simulink model "w3_warplab_trigger_proc"  (Simulink 7.7)
settings: Solver=ode45  StartTime=0.0  StopTime=60  RelTol=1e-3
InitFcn:
  | w3_warplab_trigger_proc_init
StartFcn:
  | w3_warplab_trigger_proc_init
undefined symbols (not defined in the file): gcbh, xlBlockLoadCallback, xlGetNormalizedPeriod
libraries: xbsIndex_r4 x1289, xbsEDKLib_r4 x1, simulink x1
(part 9 of 10)

== system w3_warplab_trigger_proc/Trigger Sources/Energy/AntC Detector/Busy Detection/S-R Latch ==
  R : Inport
  S : Inport  Port=2
  Constant1 : xbsIndex_r4/Constant  const=1  gui_display_data_type=Fixed-point  arith_type=Boolean  n_bits=1  bin_pt=0  preci_type=Single  exp_width=8  frac_width=24  explicit_period=off  period=1  equ=P=C  opselect=C  inp2=PCIN>>17  opr=+  inp1=P  carry=CIN  dbl_ovrd=off  block_type=constant
      settings: block_version=VER_STRING_GOES_HERE
  Register2 : xbsIndex_r4/Register  init=0  rst=on  en=on  dbl_ovrd=off  block_type=register
      settings: xl_area=[1 1 0 0 0 0 0]  block_version=VER_STRING_GOES_HERE
  Q : Outport
  wires:
  Constant1/1 -> Register2/1
  R/1 -> Register2/2
  Register2/1 -> Q/1
  S/1 -> Register2/3

== system w3_warplab_trigger_proc/Trigger Sources/Energy/AntC Detector/Idle Detection/S-R Latch ==
  R : Inport
  S : Inport  Port=2
  Constant1 : xbsIndex_r4/Constant  const=1  gui_display_data_type=Fixed-point  arith_type=Boolean  n_bits=1  bin_pt=0  preci_type=Single  exp_width=8  frac_width=24  explicit_period=off  period=1  equ=P=C  opselect=C  inp2=PCIN>>17  opr=+  inp1=P  carry=CIN  dbl_ovrd=off  block_type=constant
      settings: block_version=VER_STRING_GOES_HERE
  Register2 : xbsIndex_r4/Register  init=0  rst=on  en=on  dbl_ovrd=off  block_type=register
      settings: xl_area=[1 1 0 0 0 0 0]  block_version=VER_STRING_GOES_HERE
  Q : Outport
  wires:
  S/1 -> Register2/3
  Register2/1 -> Q/1
  R/1 -> Register2/2
  Constant1/1 -> Register2/1

== system w3_warplab_trigger_proc/Trigger Sources/Energy/AntC Detector/Running Sum/Long Reset Gen ==
  duration : Inport
  reset_in : Inport  Port=2
  Counter : xbsIndex_r4/Counter  cnt_type=Free Running  cnt_to=0  operation=Up  start_count=0  cnt_by_val=1  arith_type=Unsigned  n_bits=8  bin_pt=0  load_pin=off  rst=on  en=on  explicit_period=off  period=4  dbl_ovrd=off  use_behavioral_HDL=off  implementation=Fabric  use_rpm=off  block_type=counter
      settings: block_version=VER_STRING_GOES_HERE
  Relational : xbsIndex_r4/Relational  mode=a=b  en=off  latency=0  dbl_ovrd=off  block_type=relational
      settings: block_version=VER_STRING_GOES_HERE
  S-R Latch : Subsystem
  reset_out : Outport
  wires:
  Relational/1 -> Counter/1, S-R Latch/2(R)
  Counter/1 -> Relational/1
  reset_in/1 -> S-R Latch/1(S)
  duration/1 -> Relational/2
  S-R Latch/1(Q) -> Counter/2, reset_out/1

== system w3_warplab_trigger_proc/Trigger Sources/Energy/AntD Detector/Busy Detection/S-R Latch ==
  R : Inport
  S : Inport  Port=2
  Constant1 : xbsIndex_r4/Constant  const=1  gui_display_data_type=Fixed-point  arith_type=Boolean  n_bits=1  bin_pt=0  preci_type=Single  exp_width=8  frac_width=24  explicit_period=off  period=1  equ=P=C  opselect=C  inp2=PCIN>>17  opr=+  inp1=P  carry=CIN  dbl_ovrd=off  block_type=constant
      settings: block_version=VER_STRING_GOES_HERE
  Register2 : xbsIndex_r4/Register  init=0  rst=on  en=on  dbl_ovrd=off  block_type=register
      settings: xl_area=[1 1 0 0 0 0 0]  block_version=VER_STRING_GOES_HERE
  Q : Outport
  wires:
  Constant1/1 -> Register2/1
  R/1 -> Register2/2
  Register2/1 -> Q/1
  S/1 -> Register2/3

== system w3_warplab_trigger_proc/Trigger Sources/Energy/AntD Detector/Idle Detection/S-R Latch ==
  R : Inport
  S : Inport  Port=2
  Constant1 : xbsIndex_r4/Constant  const=1  gui_display_data_type=Fixed-point  arith_type=Boolean  n_bits=1  bin_pt=0  preci_type=Single  exp_width=8  frac_width=24  explicit_period=off  period=1  equ=P=C  opselect=C  inp2=PCIN>>17  opr=+  inp1=P  carry=CIN  dbl_ovrd=off  block_type=constant
      settings: block_version=VER_STRING_GOES_HERE
  Register2 : xbsIndex_r4/Register  init=0  rst=on  en=on  dbl_ovrd=off  block_type=register
      settings: xl_area=[1 1 0 0 0 0 0]  block_version=VER_STRING_GOES_HERE
  Q : Outport
  wires:
  S/1 -> Register2/3
  Register2/1 -> Q/1
  R/1 -> Register2/2
  Constant1/1 -> Register2/1

== system w3_warplab_trigger_proc/Trigger Sources/Energy/AntD Detector/Running Sum/Long Reset Gen ==
  duration : Inport
  reset_in : Inport  Port=2
  Counter : xbsIndex_r4/Counter  cnt_type=Free Running  cnt_to=0  operation=Up  start_count=0  cnt_by_val=1  arith_type=Unsigned  n_bits=8  bin_pt=0  load_pin=off  rst=on  en=on  explicit_period=off  period=4  dbl_ovrd=off  use_behavioral_HDL=off  implementation=Fabric  use_rpm=off  block_type=counter
      settings: block_version=VER_STRING_GOES_HERE
  Relational : xbsIndex_r4/Relational  mode=a=b  en=off  latency=0  dbl_ovrd=off  block_type=relational
      settings: block_version=VER_STRING_GOES_HERE
  S-R Latch : Subsystem
  reset_out : Outport
  wires:
  S-R Latch/1(Q) -> reset_out/1, Counter/2
  duration/1 -> Relational/2
  reset_in/1 -> S-R Latch/1(S)
  Counter/1 -> Relational/1
  Relational/1 -> S-R Latch/2(R), Counter/1

== system w3_warplab_trigger_proc/Trigger Sources/Ethernet A/Pkt Comp/Pkt Match 0/Pkt Match Fail ==
  S : Inport
  R : Inport  Port=2
  Constant5 : xbsIndex_r4/Constant  const=1  gui_display_data_type=Fixed-point  arith_type=Unsigned  n_bits=1  bin_pt=0  preci_type=Single  exp_width=8  frac_width=24  explicit_period=off  period=1  equ=P=C  opselect=C  inp2=PCIN>>17  opr=+  inp1=P  carry=CIN  dbl_ovrd=off  block_type=constant
  Convert : xbsIndex_r4/Convert  gui_display_data_type=Boolean  arith_type=Boolean  n_bits=16  bin_pt=14  float_type=Single  exp_bits=8  fraction_bits=24  quantization=Truncate  overflow=Wrap  en=off  latency=0  dbl_ovrd=off  pipeline=off  block_type=convert
  Convert1 : xbsIndex_r4/Convert  gui_display_data_type=Boolean  arith_type=Boolean  n_bits=16  bin_pt=14  float_type=Single  exp_bits=8  fraction_bits=24  quantization=Truncate  overflow=Wrap  en=off  latency=0  dbl_ovrd=off  pipeline=off  block_type=convert
  Register : xbsIndex_r4/Register  init=0  rst=on  en=on  dbl_ovrd=off  block_type=register
  Q : Outport
  wires:
  Constant5/1 -> Register/1
  R/1 -> Convert/1
  Register/1 -> Q/1
  S/1 -> Convert1/1
  Convert/1 -> Register/2
  Convert1/1 -> Register/3

== system w3_warplab_trigger_proc/Trigger Sources/Ethernet A/Pkt Comp/Word Comp 0/Byte Comp 0 ==
  note: Valid Op Codes:
      | 0: Don't care (always match)
      | 1: Equal (all bits match)
      | 2: Not-equal (>0 bits don't match)
      | 3: Any bit matches (AND(T,D)>0)
  Data : Inport
  Op : Inport  Port=2
  Template : Inport  Port=3
  2LSB : xbsIndex_r4/Slice  nbits=2  boolean_output=off  mode=Lower Bit Location + Width  bit1=0  base1=MSB of Input  bit0=0  base0=LSB of Input  dbl_ovrd=off  block_type=slice
  Any of AND : Subsystem
  Constant : xbsIndex_r4/Constant  const=1  gui_display_data_type=Boolean  arith_type=Boolean  n_bits=16  bin_pt=14  preci_type=Single  exp_width=8  frac_width=24  explicit_period=off  period=1  equ=P=C  opselect=C  inp2=PCIN>>17  opr=+  inp1=P  carry=CIN  dbl_ovrd=off  block_type=constant
  Constant1 : xbsIndex_r4/Constant  const=0  gui_display_data_type=Fixed-point  arith_type=Unsigned  n_bits=1  bin_pt=0  preci_type=Single  exp_width=8  frac_width=24  explicit_period=off  period=1  equ=P=C  opselect=C  inp2=PCIN>>17  opr=+  inp1=P  carry=CIN  dbl_ovrd=off  block_type=constant
  Constant2 : xbsIndex_r4/Constant  const=0  gui_display_data_type=Fixed-point  arith_type=Unsigned  n_bits=1  bin_pt=0  preci_type=Single  exp_width=8  frac_width=24  explicit_period=off  period=1  equ=P=C  opselect=C  inp2=PCIN>>17  opr=+  inp1=P  carry=CIN  dbl_ovrd=off  block_type=constant
  Constant3 : xbsIndex_r4/Constant  const=0  gui_display_data_type=Fixed-point  arith_type=Unsigned  n_bits=1  bin_pt=0  preci_type=Single  exp_width=8  frac_width=24  explicit_period=off  period=1  equ=P=C  opselect=C  inp2=PCIN>>17  opr=+  inp1=P  carry=CIN  dbl_ovrd=off  block_type=constant
  Constant4 : xbsIndex_r4/Constant  const=1  gui_display_data_type=Fixed-point  arith_type=Unsigned  n_bits=1  bin_pt=0  preci_type=Single  exp_width=8  frac_width=24  explicit_period=off  period=1  equ=P=C  opselect=C  inp2=PCIN>>17  opr=+  inp1=P  carry=CIN  dbl_ovrd=off  block_type=constant
  Equal : Subsystem
  Mux : xbsIndex_r4/Mux  inputs=4  en=off  latency=0  precision=Full  arith_type=Unsigned  n_bits=16  bin_pt=14  quantization=Truncate  overflow=Wrap  dbl_ovrd=off  block_type=mux
  Mux1 : xbsIndex_r4/Mux  inputs=4  en=off  latency=0  precision=Full  arith_type=Unsigned  n_bits=16  bin_pt=14  quantization=Truncate  overflow=Wrap  dbl_ovrd=off  block_type=mux
  Not Equal : Subsystem
  Res : Outport
  Or Op : Outport  Port=2
  wires:
  Op/1 -> 2LSB/1
  Mux/1 -> Res/1
  Constant/1 -> Mux/2
  Equal/1(R) -> Mux/3
  Not Equal/1(R) -> Mux/4
  Any of AND/1(R) -> Mux/5
  Data/1 -> Equal/1(D), Not Equal/1(D), Any of AND/1(D)
  Template/1 -> Equal/2(BT), Not Equal/2(BT), Any of AND/2(T)
  2LSB/1 -> Mux/1, Mux1/1
  Mux1/1 -> Or Op/1
  Constant1/1 -> Mux1/2
  Constant2/1 -> Mux1/3
  Constant3/1 -> Mux1/4
  Constant4/1 -> Mux1/5

== system w3_warplab_trigger_proc/Trigger Sources/Ethernet A/Pkt Comp/Word Comp 0/Byte Comp 1 ==
  note: Valid Op Codes:
      | 0: Don't care (always match)
      | 1: Equal (all bits match)
      | 2: Not-equal (>0 bits don't match)
      | 3: Any bit matches (AND(T,D)>0)
  Data : Inport
  Op : Inport  Port=2
  Template : Inport  Port=3
  2LSB : xbsIndex_r4/Slice  nbits=2  boolean_output=off  mode=Lower Bit Location + Width  bit1=0  base1=MSB of Input  bit0=0  base0=LSB of Input  dbl_ovrd=off  block_type=slice
  Any of AND : Subsystem
  Constant : xbsIndex_r4/Constant  const=1  gui_display_data_type=Boolean  arith_type=Boolean  n_bits=16  bin_pt=14  preci_type=Single  exp_width=8  frac_width=24  explicit_period=off  period=1  equ=P=C  opselect=C  inp2=PCIN>>17  opr=+  inp1=P  carry=CIN  dbl_ovrd=off  block_type=constant
  Constant1 : xbsIndex_r4/Constant  const=0  gui_display_data_type=Fixed-point  arith_type=Unsigned  n_bits=1  bin_pt=0  preci_type=Single  exp_width=8  frac_width=24  explicit_period=off  period=1  equ=P=C  opselect=C  inp2=PCIN>>17  opr=+  inp1=P  carry=CIN  dbl_ovrd=off  block_type=constant
  Constant2 : xbsIndex_r4/Constant  const=0  gui_display_data_type=Fixed-point  arith_type=Unsigned  n_bits=1  bin_pt=0  preci_type=Single  exp_width=8  frac_width=24  explicit_period=off  period=1  equ=P=C  opselect=C  inp2=PCIN>>17  opr=+  inp1=P  carry=CIN  dbl_ovrd=off  block_type=constant
  Constant3 : xbsIndex_r4/Constant  const=0  gui_display_data_type=Fixed-point  arith_type=Unsigned  n_bits=1  bin_pt=0  preci_type=Single  exp_width=8  frac_width=24  explicit_period=off  period=1  equ=P=C  opselect=C  inp2=PCIN>>17  opr=+  inp1=P  carry=CIN  dbl_ovrd=off  block_type=constant
  Constant4 : xbsIndex_r4/Constant  const=1  gui_display_data_type=Fixed-point  arith_type=Unsigned  n_bits=1  bin_pt=0  preci_type=Single  exp_width=8  frac_width=24  explicit_period=off  period=1  equ=P=C  opselect=C  inp2=PCIN>>17  opr=+  inp1=P  carry=CIN  dbl_ovrd=off  block_type=constant
  Equal : Subsystem
  Mux : xbsIndex_r4/Mux  inputs=4  en=off  latency=0  precision=Full  arith_type=Unsigned  n_bits=16  bin_pt=14  quantization=Truncate  overflow=Wrap  dbl_ovrd=off  block_type=mux
  Mux1 : xbsIndex_r4/Mux  inputs=4  en=off  latency=0  precision=Full  arith_type=Unsigned  n_bits=16  bin_pt=14  quantization=Truncate  overflow=Wrap  dbl_ovrd=off  block_type=mux
  Not Equal : Subsystem
  Res : Outport
  Or Op : Outport  Port=2
  wires:
  Constant4/1 -> Mux1/5
  Constant3/1 -> Mux1/4
  Constant2/1 -> Mux1/3
  Constant1/1 -> Mux1/2
  Mux1/1 -> Or Op/1
  2LSB/1 -> Mux1/1, Mux/1
  Template/1 -> Any of AND/2(T), Not Equal/2(BT), Equal/2(BT)
  Data/1 -> Any of AND/1(D), Not Equal/1(D), Equal/1(D)
  Any of AND/1(R) -> Mux/5
  Not Equal/1(R) -> Mux/4
  Equal/1(R) -> Mux/3
  Constant/1 -> Mux/2
  Mux/1 -> Res/1
  Op/1 -> 2LSB/1

== system w3_warplab_trigger_proc/Trigger Sources/Ethernet A/Pkt Comp/Word Comp 0/Byte Comp 2 ==
  note: Valid Op Codes:
      | 0: Don't care (always match)
      | 1: Equal (all bits match)
      | 2: Not-equal (>0 bits don't match)
      | 3: Any bit matches (AND(T,D)>0)
  Data : Inport
  Op : Inport  Port=2
  Template : Inport  Port=3
  2LSB : xbsIndex_r4/Slice  nbits=2  boolean_output=off  mode=Lower Bit Location + Width  bit1=0  base1=MSB of Input  bit0=0  base0=LSB of Input  dbl_ovrd=off  block_type=slice
  Any of AND : Subsystem
  Constant : xbsIndex_r4/Constant  const=1  gui_display_data_type=Boolean  arith_type=Boolean  n_bits=16  bin_pt=14  preci_type=Single  exp_width=8  frac_width=24  explicit_period=off  period=1  equ=P=C  opselect=C  inp2=PCIN>>17  opr=+  inp1=P  carry=CIN  dbl_ovrd=off  block_type=constant
  Constant1 : xbsIndex_r4/Constant  const=0  gui_display_data_type=Fixed-point  arith_type=Unsigned  n_bits=1  bin_pt=0  preci_type=Single  exp_width=8  frac_width=24  explicit_period=off  period=1  equ=P=C  opselect=C  inp2=PCIN>>17  opr=+  inp1=P  carry=CIN  dbl_ovrd=off  block_type=constant
  Constant2 : xbsIndex_r4/Constant  const=0  gui_display_data_type=Fixed-point  arith_type=Unsigned  n_bits=1  bin_pt=0  preci_type=Single  exp_width=8  frac_width=24  explicit_period=off  period=1  equ=P=C  opselect=C  inp2=PCIN>>17  opr=+  inp1=P  carry=CIN  dbl_ovrd=off  block_type=constant
  Constant3 : xbsIndex_r4/Constant  const=0  gui_display_data_type=Fixed-point  arith_type=Unsigned  n_bits=1  bin_pt=0  preci_type=Single  exp_width=8  frac_width=24  explicit_period=off  period=1  equ=P=C  opselect=C  inp2=PCIN>>17  opr=+  inp1=P  carry=CIN  dbl_ovrd=off  block_type=constant
  Constant4 : xbsIndex_r4/Constant  const=1  gui_display_data_type=Fixed-point  arith_type=Unsigned  n_bits=1  bin_pt=0  preci_type=Single  exp_width=8  frac_width=24  explicit_period=off  period=1  equ=P=C  opselect=C  inp2=PCIN>>17  opr=+  inp1=P  carry=CIN  dbl_ovrd=off  block_type=constant
  Equal : Subsystem
  Mux : xbsIndex_r4/Mux  inputs=4  en=off  latency=0  precision=Full  arith_type=Unsigned  n_bits=16  bin_pt=14  quantization=Truncate  overflow=Wrap  dbl_ovrd=off  block_type=mux
  Mux1 : xbsIndex_r4/Mux  inputs=4  en=off  latency=0  precision=Full  arith_type=Unsigned  n_bits=16  bin_pt=14  quantization=Truncate  overflow=Wrap  dbl_ovrd=off  block_type=mux
  Not Equal : Subsystem
  Res : Outport
  Or Op : Outport  Port=2
  wires:
  Op/1 -> 2LSB/1
  Mux/1 -> Res/1
  Constant/1 -> Mux/2
  Equal/1(R) -> Mux/3
  Not Equal/1(R) -> Mux/4
  Any of AND/1(R) -> Mux/5
  Data/1 -> Equal/1(D), Not Equal/1(D), Any of AND/1(D)
  Template/1 -> Equal/2(BT), Not Equal/2(BT), Any of AND/2(T)
  2LSB/1 -> Mux/1, Mux1/1
  Mux1/1 -> Or Op/1
  Constant1/1 -> Mux1/2
  Constant2/1 -> Mux1/3
  Constant3/1 -> Mux1/4
  Constant4/1 -> Mux1/5

== system w3_warplab_trigger_proc/Trigger Sources/Ethernet A/Pkt Comp/Word Comp 0/Byte Comp 3 ==
  note: Valid Op Codes:
      | 0: Don't care (always match)
      | 1: Equal (all bits match)
      | 2: Not-equal (>0 bits don't match)
      | 3: Any bit matches (AND(T,D)>0)
  Data : Inport
  Op : Inport  Port=2
  Template : Inport  Port=3
  2LSB : xbsIndex_r4/Slice  nbits=2  boolean_output=off  mode=Lower Bit Location + Width  bit1=0  base1=MSB of Input  bit0=0  base0=LSB of Input  dbl_ovrd=off  block_type=slice
  Any of AND : Subsystem
  Constant : xbsIndex_r4/Constant  const=1  gui_display_data_type=Boolean  arith_type=Boolean  n_bits=16  bin_pt=14  preci_type=Single  exp_width=8  frac_width=24  explicit_period=off  period=1  equ=P=C  opselect=C  inp2=PCIN>>17  opr=+  inp1=P  carry=CIN  dbl_ovrd=off  block_type=constant
  Constant1 : xbsIndex_r4/Constant  const=0  gui_display_data_type=Fixed-point  arith_type=Unsigned  n_bits=1  bin_pt=0  preci_type=Single  exp_width=8  frac_width=24  explicit_period=off  period=1  equ=P=C  opselect=C  inp2=PCIN>>17  opr=+  inp1=P  carry=CIN  dbl_ovrd=off  block_type=constant
  Constant2 : xbsIndex_r4/Constant  const=0  gui_display_data_type=Fixed-point  arith_type=Unsigned  n_bits=1  bin_pt=0  preci_type=Single  exp_width=8  frac_width=24  explicit_period=off  period=1  equ=P=C  opselect=C  inp2=PCIN>>17  opr=+  inp1=P  carry=CIN  dbl_ovrd=off  block_type=constant
  Constant3 : xbsIndex_r4/Constant  const=0  gui_display_data_type=Fixed-point  arith_type=Unsigned  n_bits=1  bin_pt=0  preci_type=Single  exp_width=8  frac_width=24  explicit_period=off  period=1  equ=P=C  opselect=C  inp2=PCIN>>17  opr=+  inp1=P  carry=CIN  dbl_ovrd=off  block_type=constant
  Constant4 : xbsIndex_r4/Constant  const=1  gui_display_data_type=Fixed-point  arith_type=Unsigned  n_bits=1  bin_pt=0  preci_type=Single  exp_width=8  frac_width=24  explicit_period=off  period=1  equ=P=C  opselect=C  inp2=PCIN>>17  opr=+  inp1=P  carry=CIN  dbl_ovrd=off  block_type=constant
  Equal : Subsystem
  Mux : xbsIndex_r4/Mux  inputs=4  en=off  latency=0  precision=Full  arith_type=Unsigned  n_bits=16  bin_pt=14  quantization=Truncate  overflow=Wrap  dbl_ovrd=off  block_type=mux
  Mux1 : xbsIndex_r4/Mux  inputs=4  en=off  latency=0  precision=Full  arith_type=Unsigned  n_bits=16  bin_pt=14  quantization=Truncate  overflow=Wrap  dbl_ovrd=off  block_type=mux
  Not Equal : Subsystem
  Res : Outport
  Or Op : Outport  Port=2
  wires:
  Constant4/1 -> Mux1/5
  Constant3/1 -> Mux1/4
  Constant2/1 -> Mux1/3
  Constant1/1 -> Mux1/2
  Mux1/1 -> Or Op/1
  2LSB/1 -> Mux1/1, Mux/1
  Template/1 -> Any of AND/2(T), Not Equal/2(BT), Equal/2(BT)
  Data/1 -> Any of AND/1(D), Not Equal/1(D), Equal/1(D)
  Any of AND/1(R) -> Mux/5
  Not Equal/1(R) -> Mux/4
  Equal/1(R) -> Mux/3
  Constant/1 -> Mux/2
  Mux/1 -> Res/1
  Op/1 -> 2LSB/1

== system w3_warplab_trigger_proc/Trigger Sources/Ethernet A/Pkt Comp/Word Comp 0/Subsystem ==
  32b : Inport
  8LSB+0 : xbsIndex_r4/Slice  nbits=8  boolean_output=off  mode=Lower Bit Location + Width  bit1=0  base1=MSB of Input  bit0=0  base0=LSB of Input  dbl_ovrd=off  block_type=slice
  8LSB+16 : xbsIndex_r4/Slice  nbits=8  boolean_output=off  mode=Lower Bit Location + Width  bit1=0  base1=MSB of Input  bit0=16  base0=LSB of Input  dbl_ovrd=off  block_type=slice
  8LSB+24 : xbsIndex_r4/Slice  nbits=8  boolean_output=off  mode=Lower Bit Location + Width  bit1=0  base1=MSB of Input  bit0=24  base0=LSB of Input  dbl_ovrd=off  block_type=slice
  8LSB+8 : xbsIndex_r4/Slice  nbits=8  boolean_output=off  mode=Lower Bit Location + Width  bit1=0  base1=MSB of Input  bit0=8  base0=LSB of Input  dbl_ovrd=off  block_type=slice
  B0 : Outport
  B1 : Outport  Port=2
  B2 : Outport  Port=3
  B3 : Outport  Port=4
  wires:
  32b/1 -> 8LSB+0/1, 8LSB+8/1, 8LSB+16/1, 8LSB+24/1
  8LSB+0/1 -> B0/1
  8LSB+8/1 -> B1/1
  8LSB+16/1 -> B2/1
  8LSB+24/1 -> B3/1

== system w3_warplab_trigger_proc/Trigger Sources/Ethernet A/Pkt Comp/Word Comp 0/Subsystem1 ==
  32b : Inport
  8LSB+0 : xbsIndex_r4/Slice  nbits=8  boolean_output=off  mode=Lower Bit Location + Width  bit1=0  base1=MSB of Input  bit0=0  base0=LSB of Input  dbl_ovrd=off  block_type=slice
  8LSB+16 : xbsIndex_r4/Slice  nbits=8  boolean_output=off  mode=Lower Bit Location + Width  bit1=0  base1=MSB of Input  bit0=16  base0=LSB of Input  dbl_ovrd=off  block_type=slice
  8LSB+24 : xbsIndex_r4/Slice  nbits=8  boolean_output=off  mode=Lower Bit Location + Width  bit1=0  base1=MSB of Input  bit0=24  base0=LSB of Input  dbl_ovrd=off  block_type=slice
  8LSB+8 : xbsIndex_r4/Slice  nbits=8  boolean_output=off  mode=Lower Bit Location + Width  bit1=0  base1=MSB of Input  bit0=8  base0=LSB of Input  dbl_ovrd=off  block_type=slice
  B0 : Outport
  B1 : Outport  Port=2
  B2 : Outport  Port=3
  B3 : Outport  Port=4
  wires:
  8LSB+24/1 -> B3/1
  8LSB+16/1 -> B2/1
  8LSB+8/1 -> B1/1
  8LSB+0/1 -> B0/1
  32b/1 -> 8LSB+24/1, 8LSB+16/1, 8LSB+8/1, 8LSB+0/1

== system w3_warplab_trigger_proc/Trigger Sources/Ethernet A/Pkt Comp/Word Comp 0/Subsystem2 ==
  32b : Inport
  8LSB+0 : xbsIndex_r4/Slice  nbits=8  boolean_output=off  mode=Lower Bit Location + Width  bit1=0  base1=MSB of Input  bit0=0  base0=LSB of Input  dbl_ovrd=off  block_type=slice
  8LSB+16 : xbsIndex_r4/Slice  nbits=8  boolean_output=off  mode=Lower Bit Location + Width  bit1=0  base1=MSB of Input  bit0=16  base0=LSB of Input  dbl_ovrd=off  block_type=slice
  8LSB+24 : xbsIndex_r4/Slice  nbits=8  boolean_output=off  mode=Lower Bit Location + Width  bit1=0  base1=MSB of Input  bit0=24  base0=LSB of Input  dbl_ovrd=off  block_type=slice
  8LSB+8 : xbsIndex_r4/Slice  nbits=8  boolean_output=off  mode=Lower Bit Location + Width  bit1=0  base1=MSB of Input  bit0=8  base0=LSB of Input  dbl_ovrd=off  block_type=slice
  B0 : Outport
  B1 : Outport  Port=2
  B2 : Outport  Port=3
  B3 : Outport  Port=4
  wires:
  32b/1 -> 8LSB+0/1, 8LSB+8/1, 8LSB+16/1, 8LSB+24/1
  8LSB+0/1 -> B0/1
  8LSB+8/1 -> B1/1
  8LSB+16/1 -> B2/1
  8LSB+24/1 -> B3/1

== system w3_warplab_trigger_proc/Trigger Sources/Ethernet B/Pkt Comp/Pkt Match 1/Pkt Match Fail ==
  S : Inport
  R : Inport  Port=2
  Constant5 : xbsIndex_r4/Constant  const=1  gui_display_data_type=Fixed-point  arith_type=Unsigned  n_bits=1  bin_pt=0  preci_type=Single  exp_width=8  frac_width=24  explicit_period=off  period=1  equ=P=C  opselect=C  inp2=PCIN>>17  opr=+  inp1=P  carry=CIN  dbl_ovrd=off  block_type=constant
  Convert : xbsIndex_r4/Convert  gui_display_data_type=Boolean  arith_type=Boolean  n_bits=16  bin_pt=14  float_type=Single  exp_bits=8  fraction_bits=24  quantization=Truncate  overflow=Wrap  en=off  latency=0  dbl_ovrd=off  pipeline=off  block_type=convert
  Convert1 : xbsIndex_r4/Convert  gui_display_data_type=Boolean  arith_type=Boolean  n_bits=16  bin_pt=14  float_type=Single  exp_bits=8  fraction_bits=24  quantization=Truncate  overflow=Wrap  en=off  latency=0  dbl_ovrd=off  pipeline=off  block_type=convert
  Register : xbsIndex_r4/Register  init=0  rst=on  en=on  dbl_ovrd=off  block_type=register
  Q : Outport
  wires:
  Constant5/1 -> Register/1
  R/1 -> Convert/1
  Register/1 -> Q/1
  S/1 -> Convert1/1
  Convert/1 -> Register/2
  Convert1/1 -> Register/3

== system w3_warplab_trigger_proc/Trigger Sources/Ethernet B/Pkt Comp/Word Comp 1/Byte Comp 0 ==
  note: Valid Op Codes:
      | 0: Don't care (always match)
      | 1: Equal (all bits match)
      | 2: Not-equal (>0 bits don't match)
      | 3: Any bit matches (AND(T,D)>0)
  Data : Inport
  Op : Inport  Port=2
  Template : Inport  Port=3
  2LSB : xbsIndex_r4/Slice  nbits=2  boolean_output=off  mode=Lower Bit Location + Width  bit1=0  base1=MSB of Input  bit0=0  base0=LSB of Input  dbl_ovrd=off  block_type=slice
  Any of AND : Subsystem
  Constant : xbsIndex_r4/Constant  const=1  gui_display_data_type=Boolean  arith_type=Boolean  n_bits=16  bin_pt=14  preci_type=Single  exp_width=8  frac_width=24  explicit_period=off  period=1  equ=P=C  opselect=C  inp2=PCIN>>17  opr=+  inp1=P  carry=CIN  dbl_ovrd=off  block_type=constant
  Constant1 : xbsIndex_r4/Constant  const=0  gui_display_data_type=Fixed-point  arith_type=Unsigned  n_bits=1  bin_pt=0  preci_type=Single  exp_width=8  frac_width=24  explicit_period=off  period=1  equ=P=C  opselect=C  inp2=PCIN>>17  opr=+  inp1=P  carry=CIN  dbl_ovrd=off  block_type=constant
  Constant2 : xbsIndex_r4/Constant  const=0  gui_display_data_type=Fixed-point  arith_type=Unsigned  n_bits=1  bin_pt=0  preci_type=Single  exp_width=8  frac_width=24  explicit_period=off  period=1  equ=P=C  opselect=C  inp2=PCIN>>17  opr=+  inp1=P  carry=CIN  dbl_ovrd=off  block_type=constant
  Constant3 : xbsIndex_r4/Constant  const=0  gui_display_data_type=Fixed-point  arith_type=Unsigned  n_bits=1  bin_pt=0  preci_type=Single  exp_width=8  frac_width=24  explicit_period=off  period=1  equ=P=C  opselect=C  inp2=PCIN>>17  opr=+  inp1=P  carry=CIN  dbl_ovrd=off  block_type=constant
  Constant4 : xbsIndex_r4/Constant  const=1  gui_display_data_type=Fixed-point  arith_type=Unsigned  n_bits=1  bin_pt=0  preci_type=Single  exp_width=8  frac_width=24  explicit_period=off  period=1  equ=P=C  opselect=C  inp2=PCIN>>17  opr=+  inp1=P  carry=CIN  dbl_ovrd=off  block_type=constant
  Equal : Subsystem
  Mux : xbsIndex_r4/Mux  inputs=4  en=off  latency=0  precision=Full  arith_type=Unsigned  n_bits=16  bin_pt=14  quantization=Truncate  overflow=Wrap  dbl_ovrd=off  block_type=mux
  Mux1 : xbsIndex_r4/Mux  inputs=4  en=off  latency=0  precision=Full  arith_type=Unsigned  n_bits=16  bin_pt=14  quantization=Truncate  overflow=Wrap  dbl_ovrd=off  block_type=mux
  Not Equal : Subsystem
  Res : Outport
  Or Op : Outport  Port=2
  wires:
  Op/1 -> 2LSB/1
  Mux/1 -> Res/1
  Constant/1 -> Mux/2
  Equal/1(R) -> Mux/3
  Not Equal/1(R) -> Mux/4
  Any of AND/1(R) -> Mux/5
  Data/1 -> Equal/1(D), Not Equal/1(D), Any of AND/1(D)
  Template/1 -> Equal/2(BT), Not Equal/2(BT), Any of AND/2(T)
  2LSB/1 -> Mux/1, Mux1/1
  Mux1/1 -> Or Op/1
  Constant1/1 -> Mux1/2
  Constant2/1 -> Mux1/3
  Constant3/1 -> Mux1/4
  Constant4/1 -> Mux1/5

== system w3_warplab_trigger_proc/Trigger Sources/Ethernet B/Pkt Comp/Word Comp 1/Byte Comp 1 ==
  note: Valid Op Codes:
      | 0: Don't care (always match)
      | 1: Equal (all bits match)
      | 2: Not-equal (>0 bits don't match)
      | 3: Any bit matches (AND(T,D)>0)
  Data : Inport
  Op : Inport  Port=2
  Template : Inport  Port=3
  2LSB : xbsIndex_r4/Slice  nbits=2  boolean_output=off  mode=Lower Bit Location + Width  bit1=0  base1=MSB of Input  bit0=0  base0=LSB of Input  dbl_ovrd=off  block_type=slice
  Any of AND : Subsystem
  Constant : xbsIndex_r4/Constant  const=1  gui_display_data_type=Boolean  arith_type=Boolean  n_bits=16  bin_pt=14  preci_type=Single  exp_width=8  frac_width=24  explicit_period=off  period=1  equ=P=C  opselect=C  inp2=PCIN>>17  opr=+  inp1=P  carry=CIN  dbl_ovrd=off  block_type=constant
  Constant1 : xbsIndex_r4/Constant  const=0  gui_display_data_type=Fixed-point  arith_type=Unsigned  n_bits=1  bin_pt=0  preci_type=Single  exp_width=8  frac_width=24  explicit_period=off  period=1  equ=P=C  opselect=C  inp2=PCIN>>17  opr=+  inp1=P  carry=CIN  dbl_ovrd=off  block_type=constant
  Constant2 : xbsIndex_r4/Constant  const=0  gui_display_data_type=Fixed-point  arith_type=Unsigned  n_bits=1  bin_pt=0  preci_type=Single  exp_width=8  frac_width=24  explicit_period=off  period=1  equ=P=C  opselect=C  inp2=PCIN>>17  opr=+  inp1=P  carry=CIN  dbl_ovrd=off  block_type=constant
  Constant3 : xbsIndex_r4/Constant  const=0  gui_display_data_type=Fixed-point  arith_type=Unsigned  n_bits=1  bin_pt=0  preci_type=Single  exp_width=8  frac_width=24  explicit_period=off  period=1  equ=P=C  opselect=C  inp2=PCIN>>17  opr=+  inp1=P  carry=CIN  dbl_ovrd=off  block_type=constant
  Constant4 : xbsIndex_r4/Constant  const=1  gui_display_data_type=Fixed-point  arith_type=Unsigned  n_bits=1  bin_pt=0  preci_type=Single  exp_width=8  frac_width=24  explicit_period=off  period=1  equ=P=C  opselect=C  inp2=PCIN>>17  opr=+  inp1=P  carry=CIN  dbl_ovrd=off  block_type=constant
  Equal : Subsystem
  Mux : xbsIndex_r4/Mux  inputs=4  en=off  latency=0  precision=Full  arith_type=Unsigned  n_bits=16  bin_pt=14  quantization=Truncate  overflow=Wrap  dbl_ovrd=off  block_type=mux
  Mux1 : xbsIndex_r4/Mux  inputs=4  en=off  latency=0  precision=Full  arith_type=Unsigned  n_bits=16  bin_pt=14  quantization=Truncate  overflow=Wrap  dbl_ovrd=off  block_type=mux
  Not Equal : Subsystem
  Res : Outport
  Or Op : Outport  Port=2
  wires:
  Constant4/1 -> Mux1/5
  Constant3/1 -> Mux1/4
  Constant2/1 -> Mux1/3
  Constant1/1 -> Mux1/2
  Mux1/1 -> Or Op/1
  2LSB/1 -> Mux1/1, Mux/1
  Template/1 -> Any of AND/2(T), Not Equal/2(BT), Equal/2(BT)
  Data/1 -> Any of AND/1(D), Not Equal/1(D), Equal/1(D)
  Any of AND/1(R) -> Mux/5
  Not Equal/1(R) -> Mux/4
  Equal/1(R) -> Mux/3
  Constant/1 -> Mux/2
  Mux/1 -> Res/1
  Op/1 -> 2LSB/1

== system w3_warplab_trigger_proc/Trigger Sources/Ethernet B/Pkt Comp/Word Comp 1/Byte Comp 2 ==
  note: Valid Op Codes:
      | 0: Don't care (always match)
      | 1: Equal (all bits match)
      | 2: Not-equal (>0 bits don't match)
      | 3: Any bit matches (AND(T,D)>0)
  Data : Inport
  Op : Inport  Port=2
  Template : Inport  Port=3
  2LSB : xbsIndex_r4/Slice  nbits=2  boolean_output=off  mode=Lower Bit Location + Width  bit1=0  base1=MSB of Input  bit0=0  base0=LSB of Input  dbl_ovrd=off  block_type=slice
  Any of AND : Subsystem
  Constant : xbsIndex_r4/Constant  const=1  gui_display_data_type=Boolean  arith_type=Boolean  n_bits=16  bin_pt=14  preci_type=Single  exp_width=8  frac_width=24  explicit_period=off  period=1  equ=P=C  opselect=C  inp2=PCIN>>17  opr=+  inp1=P  carry=CIN  dbl_ovrd=off  block_type=constant
  Constant1 : xbsIndex_r4/Constant  const=0  gui_display_data_type=Fixed-point  arith_type=Unsigned  n_bits=1  bin_pt=0  preci_type=Single  exp_width=8  frac_width=24  explicit_period=off  period=1  equ=P=C  opselect=C  inp2=PCIN>>17  opr=+  inp1=P  carry=CIN  dbl_ovrd=off  block_type=constant
  Constant2 : xbsIndex_r4/Constant  const=0  gui_display_data_type=Fixed-point  arith_type=Unsigned  n_bits=1  bin_pt=0  preci_type=Single  exp_width=8  frac_width=24  explicit_period=off  period=1  equ=P=C  opselect=C  inp2=PCIN>>17  opr=+  inp1=P  carry=CIN  dbl_ovrd=off  block_type=constant
  Constant3 : xbsIndex_r4/Constant  const=0  gui_display_data_type=Fixed-point  arith_type=Unsigned  n_bits=1  bin_pt=0  preci_type=Single  exp_width=8  frac_width=24  explicit_period=off  period=1  equ=P=C  opselect=C  inp2=PCIN>>17  opr=+  inp1=P  carry=CIN  dbl_ovrd=off  block_type=constant
  Constant4 : xbsIndex_r4/Constant  const=1  gui_display_data_type=Fixed-point  arith_type=Unsigned  n_bits=1  bin_pt=0  preci_type=Single  exp_width=8  frac_width=24  explicit_period=off  period=1  equ=P=C  opselect=C  inp2=PCIN>>17  opr=+  inp1=P  carry=CIN  dbl_ovrd=off  block_type=constant
  Equal : Subsystem
  Mux : xbsIndex_r4/Mux  inputs=4  en=off  latency=0  precision=Full  arith_type=Unsigned  n_bits=16  bin_pt=14  quantization=Truncate  overflow=Wrap  dbl_ovrd=off  block_type=mux
  Mux1 : xbsIndex_r4/Mux  inputs=4  en=off  latency=0  precision=Full  arith_type=Unsigned  n_bits=16  bin_pt=14  quantization=Truncate  overflow=Wrap  dbl_ovrd=off  block_type=mux
  Not Equal : Subsystem
  Res : Outport
  Or Op : Outport  Port=2
  wires:
  Op/1 -> 2LSB/1
  Mux/1 -> Res/1
  Constant/1 -> Mux/2
  Equal/1(R) -> Mux/3
  Not Equal/1(R) -> Mux/4
  Any of AND/1(R) -> Mux/5
  Data/1 -> Equal/1(D), Not Equal/1(D), Any of AND/1(D)
  Template/1 -> Equal/2(BT), Not Equal/2(BT), Any of AND/2(T)
  2LSB/1 -> Mux/1, Mux1/1
  Mux1/1 -> Or Op/1
  Constant1/1 -> Mux1/2
  Constant2/1 -> Mux1/3
  Constant3/1 -> Mux1/4
  Constant4/1 -> Mux1/5

== system w3_warplab_trigger_proc/Trigger Sources/Ethernet B/Pkt Comp/Word Comp 1/Byte Comp 3 ==
  note: Valid Op Codes:
      | 0: Don't care (always match)
      | 1: Equal (all bits match)
      | 2: Not-equal (>0 bits don't match)
      | 3: Any bit matches (AND(T,D)>0)
  Data : Inport
  Op : Inport  Port=2
  Template : Inport  Port=3
  2LSB : xbsIndex_r4/Slice  nbits=2  boolean_output=off  mode=Lower Bit Location + Width  bit1=0  base1=MSB of Input  bit0=0  base0=LSB of Input  dbl_ovrd=off  block_type=slice
  Any of AND : Subsystem
  Constant : xbsIndex_r4/Constant  const=1  gui_display_data_type=Boolean  arith_type=Boolean  n_bits=16  bin_pt=14  preci_type=Single  exp_width=8  frac_width=24  explicit_period=off  period=1  equ=P=C  opselect=C  inp2=PCIN>>17  opr=+  inp1=P  carry=CIN  dbl_ovrd=off  block_type=constant
  Constant1 : xbsIndex_r4/Constant  const=0  gui_display_data_type=Fixed-point  arith_type=Unsigned  n_bits=1  bin_pt=0  preci_type=Single  exp_width=8  frac_width=24  explicit_period=off  period=1  equ=P=C  opselect=C  inp2=PCIN>>17  opr=+  inp1=P  carry=CIN  dbl_ovrd=off  block_type=constant
  Constant2 : xbsIndex_r4/Constant  const=0  gui_display_data_type=Fixed-point  arith_type=Unsigned  n_bits=1  bin_pt=0  preci_type=Single  exp_width=8  frac_width=24  explicit_period=off  period=1  equ=P=C  opselect=C  inp2=PCIN>>17  opr=+  inp1=P  carry=CIN  dbl_ovrd=off  block_type=constant
  Constant3 : xbsIndex_r4/Constant  const=0  gui_display_data_type=Fixed-point  arith_type=Unsigned  n_bits=1  bin_pt=0  preci_type=Single  exp_width=8  frac_width=24  explicit_period=off  period=1  equ=P=C  opselect=C  inp2=PCIN>>17  opr=+  inp1=P  carry=CIN  dbl_ovrd=off  block_type=constant
  Constant4 : xbsIndex_r4/Constant  const=1  gui_display_data_type=Fixed-point  arith_type=Unsigned  n_bits=1  bin_pt=0  preci_type=Single  exp_width=8  frac_width=24  explicit_period=off  period=1  equ=P=C  opselect=C  inp2=PCIN>>17  opr=+  inp1=P  carry=CIN  dbl_ovrd=off  block_type=constant
  Equal : Subsystem
  Mux : xbsIndex_r4/Mux  inputs=4  en=off  latency=0  precision=Full  arith_type=Unsigned  n_bits=16  bin_pt=14  quantization=Truncate  overflow=Wrap  dbl_ovrd=off  block_type=mux
  Mux1 : xbsIndex_r4/Mux  inputs=4  en=off  latency=0  precision=Full  arith_type=Unsigned  n_bits=16  bin_pt=14  quantization=Truncate  overflow=Wrap  dbl_ovrd=off  block_type=mux
  Not Equal : Subsystem
  Res : Outport
  Or Op : Outport  Port=2
  wires:
  Constant4/1 -> Mux1/5
  Constant3/1 -> Mux1/4
  Constant2/1 -> Mux1/3
  Constant1/1 -> Mux1/2
  Mux1/1 -> Or Op/1
  2LSB/1 -> Mux1/1, Mux/1
  Template/1 -> Any of AND/2(T), Not Equal/2(BT), Equal/2(BT)
  Data/1 -> Any of AND/1(D), Not Equal/1(D), Equal/1(D)
  Any of AND/1(R) -> Mux/5
  Not Equal/1(R) -> Mux/4
  Equal/1(R) -> Mux/3
  Constant/1 -> Mux/2
  Mux/1 -> Res/1
  Op/1 -> 2LSB/1

== system w3_warplab_trigger_proc/Trigger Sources/Ethernet B/Pkt Comp/Word Comp 1/Subsystem ==
  32b : Inport
  8LSB+0 : xbsIndex_r4/Slice  nbits=8  boolean_output=off  mode=Lower Bit Location + Width  bit1=0  base1=MSB of Input  bit0=0  base0=LSB of Input  dbl_ovrd=off  block_type=slice
  8LSB+16 : xbsIndex_r4/Slice  nbits=8  boolean_output=off  mode=Lower Bit Location + Width  bit1=0  base1=MSB of Input  bit0=16  base0=LSB of Input  dbl_ovrd=off  block_type=slice
  8LSB+24 : xbsIndex_r4/Slice  nbits=8  boolean_output=off  mode=Lower Bit Location + Width  bit1=0  base1=MSB of Input  bit0=24  base0=LSB of Input  dbl_ovrd=off  block_type=slice
  8LSB+8 : xbsIndex_r4/Slice  nbits=8  boolean_output=off  mode=Lower Bit Location + Width  bit1=0  base1=MSB of Input  bit0=8  base0=LSB of Input  dbl_ovrd=off  block_type=slice
  B0 : Outport
  B1 : Outport  Port=2
  B2 : Outport  Port=3
  B3 : Outport  Port=4
  wires:
  32b/1 -> 8LSB+0/1, 8LSB+8/1, 8LSB+16/1, 8LSB+24/1
  8LSB+0/1 -> B0/1
  8LSB+8/1 -> B1/1
  8LSB+16/1 -> B2/1
  8LSB+24/1 -> B3/1

== system w3_warplab_trigger_proc/Trigger Sources/Ethernet B/Pkt Comp/Word Comp 1/Subsystem1 ==
  32b : Inport
  8LSB+0 : xbsIndex_r4/Slice  nbits=8  boolean_output=off  mode=Lower Bit Location + Width  bit1=0  base1=MSB of Input  bit0=0  base0=LSB of Input  dbl_ovrd=off  block_type=slice
  8LSB+16 : xbsIndex_r4/Slice  nbits=8  boolean_output=off  mode=Lower Bit Location + Width  bit1=0  base1=MSB of Input  bit0=16  base0=LSB of Input  dbl_ovrd=off  block_type=slice
  8LSB+24 : xbsIndex_r4/Slice  nbits=8  boolean_output=off  mode=Lower Bit Location + Width  bit1=0  base1=MSB of Input  bit0=24  base0=LSB of Input  dbl_ovrd=off  block_type=slice
  8LSB+8 : xbsIndex_r4/Slice  nbits=8  boolean_output=off  mode=Lower Bit Location + Width  bit1=0  base1=MSB of Input  bit0=8  base0=LSB of Input  dbl_ovrd=off  block_type=slice
  B0 : Outport
  B1 : Outport  Port=2
  B2 : Outport  Port=3
  B3 : Outport  Port=4
  wires:
  8LSB+24/1 -> B3/1
  8LSB+16/1 -> B2/1
  8LSB+8/1 -> B1/1
  8LSB+0/1 -> B0/1
  32b/1 -> 8LSB+24/1, 8LSB+16/1, 8LSB+8/1, 8LSB+0/1

== system w3_warplab_trigger_proc/Trigger Sources/Ethernet B/Pkt Comp/Word Comp 1/Subsystem2 ==
  32b : Inport
  8LSB+0 : xbsIndex_r4/Slice  nbits=8  boolean_output=off  mode=Lower Bit Location + Width  bit1=0  base1=MSB of Input  bit0=0  base0=LSB of Input  dbl_ovrd=off  block_type=slice
  8LSB+16 : xbsIndex_r4/Slice  nbits=8  boolean_output=off  mode=Lower Bit Location + Width  bit1=0  base1=MSB of Input  bit0=16  base0=LSB of Input  dbl_ovrd=off  block_type=slice
  8LSB+24 : xbsIndex_r4/Slice  nbits=8  boolean_output=off  mode=Lower Bit Location + Width  bit1=0  base1=MSB of Input  bit0=24  base0=LSB of Input  dbl_ovrd=off  block_type=slice
  8LSB+8 : xbsIndex_r4/Slice  nbits=8  boolean_output=off  mode=Lower Bit Location + Width  bit1=0  base1=MSB of Input  bit0=8  base0=LSB of Input  dbl_ovrd=off  block_type=slice
  B0 : Outport
  B1 : Outport  Port=2
  B2 : Outport  Port=3
  B3 : Outport  Port=4
  wires:
  32b/1 -> 8LSB+0/1, 8LSB+8/1, 8LSB+16/1, 8LSB+24/1
  8LSB+0/1 -> B0/1
  8LSB+8/1 -> B1/1
  8LSB+16/1 -> B2/1
  8LSB+24/1 -> B3/1

== system w3_warplab_trigger_proc/Trigger Sources/Energy/AntA Detector/Running Sum/Long Reset Gen/S-R Latch ==
  S : Inport
  R : Inport  Port=2
  Constant1 : xbsIndex_r4/Constant  const=1  gui_display_data_type=Fixed-point  arith_type=Boolean  n_bits=1  bin_pt=0  preci_type=Single  exp_width=8  frac_width=24  explicit_period=off  period=1  equ=P=C  opselect=C  inp2=PCIN>>17  opr=+  inp1=P  carry=CIN  dbl_ovrd=off  block_type=constant
      settings: block_version=VER_STRING_GOES_HERE
  Register2 : xbsIndex_r4/Register  init=0  rst=on  en=on  dbl_ovrd=off  block_type=register
      settings: xl_area=[1 1 0 0 0 0 0]  block_version=VER_STRING_GOES_HERE
  Q : Outport
  wires:
  Constant1/1 -> Register2/1
  R/1 -> Register2/2
  Register2/1 -> Q/1
  S/1 -> Register2/3

== system w3_warplab_trigger_proc/Trigger Sources/Energy/AntB Detector/Running Sum/Long Reset Gen/S-R Latch ==
  S : Inport
  R : Inport  Port=2
  Constant1 : xbsIndex_r4/Constant  const=1  gui_display_data_type=Fixed-point  arith_type=Boolean  n_bits=1  bin_pt=0  preci_type=Single  exp_width=8  frac_width=24  explicit_period=off  period=1  equ=P=C  opselect=C  inp2=PCIN>>17  opr=+  inp1=P  carry=CIN  dbl_ovrd=off  block_type=constant
      settings: block_version=VER_STRING_GOES_HERE
  Register2 : xbsIndex_r4/Register  init=0  rst=on  en=on  dbl_ovrd=off  block_type=register
      settings: xl_area=[1 1 0 0 0 0 0]  block_version=VER_STRING_GOES_HERE
  Q : Outport
  wires:
  S/1 -> Register2/3
  Register2/1 -> Q/1
  R/1 -> Register2/2
  Constant1/1 -> Register2/1

== system w3_warplab_trigger_proc/Trigger Sources/Energy/AntC Detector/Running Sum/Long Reset Gen/S-R Latch ==
  S : Inport
  R : Inport  Port=2
  Constant1 : xbsIndex_r4/Constant  const=1  gui_display_data_type=Fixed-point  arith_type=Boolean  n_bits=1  bin_pt=0  preci_type=Single  exp_width=8  frac_width=24  explicit_period=off  period=1  equ=P=C  opselect=C  inp2=PCIN>>17  opr=+  inp1=P  carry=CIN  dbl_ovrd=off  block_type=constant
      settings: block_version=VER_STRING_GOES_HERE
  Register2 : xbsIndex_r4/Register  init=0  rst=on  en=on  dbl_ovrd=off  block_type=register
      settings: xl_area=[1 1 0 0 0 0 0]  block_version=VER_STRING_GOES_HERE
  Q : Outport
  wires:
  Constant1/1 -> Register2/1
  R/1 -> Register2/2
  Register2/1 -> Q/1
  S/1 -> Register2/3

== system w3_warplab_trigger_proc/Trigger Sources/Energy/AntD Detector/Running Sum/Long Reset Gen/S-R Latch ==
  S : Inport
  R : Inport  Port=2
  Constant1 : xbsIndex_r4/Constant  const=1  gui_display_data_type=Fixed-point  arith_type=Boolean  n_bits=1  bin_pt=0  preci_type=Single  exp_width=8  frac_width=24  explicit_period=off  period=1  equ=P=C  opselect=C  inp2=PCIN>>17  opr=+  inp1=P  carry=CIN  dbl_ovrd=off  block_type=constant
      settings: block_version=VER_STRING_GOES_HERE
  Register2 : xbsIndex_r4/Register  init=0  rst=on  en=on  dbl_ovrd=off  block_type=register
      settings: xl_area=[1 1 0 0 0 0 0]  block_version=VER_STRING_GOES_HERE
  Q : Outport
  wires:
  S/1 -> Register2/3
  Register2/1 -> Q/1
  R/1 -> Register2/2
  Constant1/1 -> Register2/1

== system w3_warplab_trigger_proc/Trigger Sources/Ethernet A/Pkt Comp/Word Comp 0/Byte Comp 0/Any of AND ==
  D : Inport
  T : Inport  Port=2
  Constant3 : xbsIndex_r4/Constant  const=0  gui_display_data_type=Fixed-point  arith_type=Unsigned  n_bits=8  bin_pt=0  preci_type=Single  exp_width=8  frac_width=24  explicit_period=off  period=1  equ=P=C  opselect=C  inp2=PCIN>>17  opr=+  inp1=P  carry=CIN  dbl_ovrd=off  block_type=constant
  Logical : xbsIndex_r4/Logical  logical_function=AND  inputs=2  en=off  latency=0  precision=Full  arith_type=Unsigned  n_bits=16  bin_pt=0  align_bp=on  dbl_ovrd=off  block_type=logical
  Relational1 : xbsIndex_r4/Relational  mode=a!=b  en=off  latency=0  dbl_ovrd=off  block_type=relational
  R : Outport
  wires:
  Constant3/1 -> Relational1/1
  Logical/1 -> Relational1/2
  D/1 -> Logical/1
  T/1 -> Logical/2
  Relational1/1 -> R/1

== system w3_warplab_trigger_proc/Trigger Sources/Ethernet A/Pkt Comp/Word Comp 0/Byte Comp 0/Equal ==
  D : Inport
  BT : Inport  Port=2
  Relational : xbsIndex_r4/Relational  mode=a=b  en=off  latency=0  dbl_ovrd=off  block_type=relational
  R : Outport
  wires:
  D/1 -> Relational/1
  BT/1 -> Relational/2
  Relational/1 -> R/1

== system w3_warplab_trigger_proc/Trigger Sources/Ethernet A/Pkt Comp/Word Comp 0/Byte Comp 0/Not Equal ==
  D : Inport
  BT : Inport  Port=2
  Relational : xbsIndex_r4/Relational  mode=a!=b  en=off  latency=0  dbl_ovrd=off  block_type=relational
  R : Outport
  wires:
  Relational/1 -> R/1
  BT/1 -> Relational/2
  D/1 -> Relational/1

== system w3_warplab_trigger_proc/Trigger Sources/Ethernet A/Pkt Comp/Word Comp 0/Byte Comp 1/Any of AND ==
  D : Inport
  T : Inport  Port=2
  Constant3 : xbsIndex_r4/Constant  const=0  gui_display_data_type=Fixed-point  arith_type=Unsigned  n_bits=8  bin_pt=0  preci_type=Single  exp_width=8  frac_width=24  explicit_period=off  period=1  equ=P=C  opselect=C  inp2=PCIN>>17  opr=+  inp1=P  carry=CIN  dbl_ovrd=off  block_type=constant
  Logical : xbsIndex_r4/Logical  logical_function=AND  inputs=2  en=off  latency=0  precision=Full  arith_type=Unsigned  n_bits=16  bin_pt=0  align_bp=on  dbl_ovrd=off  block_type=logical
  Relational1 : xbsIndex_r4/Relational  mode=a!=b  en=off  latency=0  dbl_ovrd=off  block_type=relational
  R : Outport
  wires:
  Relational1/1 -> R/1
  T/1 -> Logical/2
  D/1 -> Logical/1
  Logical/1 -> Relational1/2
  Constant3/1 -> Relational1/1

== system w3_warplab_trigger_proc/Trigger Sources/Ethernet A/Pkt Comp/Word Comp 0/Byte Comp 1/Equal ==
  D : Inport
  BT : Inport  Port=2
  Relational : xbsIndex_r4/Relational  mode=a=b  en=off  latency=0  dbl_ovrd=off  block_type=relational
  R : Outport
  wires:
  Relational/1 -> R/1
  BT/1 -> Relational/2
  D/1 -> Relational/1

== system w3_warplab_trigger_proc/Trigger Sources/Ethernet A/Pkt Comp/Word Comp 0/Byte Comp 1/Not Equal ==
  D : Inport
  BT : Inport  Port=2
  Relational : xbsIndex_r4/Relational  mode=a!=b  en=off  latency=0  dbl_ovrd=off  block_type=relational
  R : Outport
  wires:
  D/1 -> Relational/1
  BT/1 -> Relational/2
  Relational/1 -> R/1

== system w3_warplab_trigger_proc/Trigger Sources/Ethernet A/Pkt Comp/Word Comp 0/Byte Comp 2/Any of AND ==
  D : Inport
  T : Inport  Port=2
  Constant3 : xbsIndex_r4/Constant  const=0  gui_display_data_type=Fixed-point  arith_type=Unsigned  n_bits=8  bin_pt=0  preci_type=Single  exp_width=8  frac_width=24  explicit_period=off  period=1  equ=P=C  opselect=C  inp2=PCIN>>17  opr=+  inp1=P  carry=CIN  dbl_ovrd=off  block_type=constant
  Logical : xbsIndex_r4/Logical  logical_function=AND  inputs=2  en=off  latency=0  precision=Full  arith_type=Unsigned  n_bits=16  bin_pt=0  align_bp=on  dbl_ovrd=off  block_type=logical
  Relational1 : xbsIndex_r4/Relational  mode=a!=b  en=off  latency=0  dbl_ovrd=off  block_type=relational
  R : Outport
  wires:
  Constant3/1 -> Relational1/1
  Logical/1 -> Relational1/2
  D/1 -> Logical/1
  T/1 -> Logical/2
  Relational1/1 -> R/1

== system w3_warplab_trigger_proc/Trigger Sources/Ethernet A/Pkt Comp/Word Comp 0/Byte Comp 2/Equal ==
  D : Inport
  BT : Inport  Port=2
  Relational : xbsIndex_r4/Relational  mode=a=b  en=off  latency=0  dbl_ovrd=off  block_type=relational
  R : Outport
  wires:
  D/1 -> Relational/1
  BT/1 -> Relational/2
  Relational/1 -> R/1

== system w3_warplab_trigger_proc/Trigger Sources/Ethernet A/Pkt Comp/Word Comp 0/Byte Comp 2/Not Equal ==
  D : Inport
  BT : Inport  Port=2
  Relational : xbsIndex_r4/Relational  mode=a!=b  en=off  latency=0  dbl_ovrd=off  block_type=relational
  R : Outport
  wires:
  Relational/1 -> R/1
  BT/1 -> Relational/2
  D/1 -> Relational/1

== system w3_warplab_trigger_proc/Trigger Sources/Ethernet A/Pkt Comp/Word Comp 0/Byte Comp 3/Any of AND ==
  D : Inport
  T : Inport  Port=2
  Constant3 : xbsIndex_r4/Constant  const=0  gui_display_data_type=Fixed-point  arith_type=Unsigned  n_bits=8  bin_pt=0  preci_type=Single  exp_width=8  frac_width=24  explicit_period=off  period=1  equ=P=C  opselect=C  inp2=PCIN>>17  opr=+  inp1=P  carry=CIN  dbl_ovrd=off  block_type=constant
  Logical : xbsIndex_r4/Logical  logical_function=AND  inputs=2  en=off  latency=0  precision=Full  arith_type=Unsigned  n_bits=16  bin_pt=0  align_bp=on  dbl_ovrd=off  block_type=logical
  Relational1 : xbsIndex_r4/Relational  mode=a!=b  en=off  latency=0  dbl_ovrd=off  block_type=relational
  R : Outport
  wires:
  Relational1/1 -> R/1
  T/1 -> Logical/2
  D/1 -> Logical/1
  Logical/1 -> Relational1/2
  Constant3/1 -> Relational1/1

== system w3_warplab_trigger_proc/Trigger Sources/Ethernet A/Pkt Comp/Word Comp 0/Byte Comp 3/Equal ==
  D : Inport
  BT : Inport  Port=2
  Relational : xbsIndex_r4/Relational  mode=a=b  en=off  latency=0  dbl_ovrd=off  block_type=relational
  R : Outport
  wires:
  Relational/1 -> R/1
  BT/1 -> Relational/2
  D/1 -> Relational/1

== system w3_warplab_trigger_proc/Trigger Sources/Ethernet A/Pkt Comp/Word Comp 0/Byte Comp 3/Not Equal ==
  D : Inport
  BT : Inport  Port=2
  Relational : xbsIndex_r4/Relational  mode=a!=b  en=off  latency=0  dbl_ovrd=off  block_type=relational
  R : Outport
  wires:
  D/1 -> Relational/1
  BT/1 -> Relational/2
  Relational/1 -> R/1

== system w3_warplab_trigger_proc/Trigger Sources/Ethernet B/Pkt Comp/Word Comp 1/Byte Comp 0/Any of AND ==
  D : Inport
  T : Inport  Port=2
  Constant3 : xbsIndex_r4/Constant  const=0  gui_display_data_type=Fixed-point  arith_type=Unsigned  n_bits=8  bin_pt=0  preci_type=Single  exp_width=8  frac_width=24  explicit_period=off  period=1  equ=P=C  opselect=C  inp2=PCIN>>17  opr=+  inp1=P  carry=CIN  dbl_ovrd=off  block_type=constant
  Logical : xbsIndex_r4/Logical  logical_function=AND  inputs=2  en=off  latency=0  precision=Full  arith_type=Unsigned  n_bits=16  bin_pt=0  align_bp=on  dbl_ovrd=off  block_type=logical
  Relational1 : xbsIndex_r4/Relational  mode=a!=b  en=off  latency=0  dbl_ovrd=off  block_type=relational
  R : Outport
  wires:
  Constant3/1 -> Relational1/1
  Logical/1 -> Relational1/2
  D/1 -> Logical/1
  T/1 -> Logical/2
  Relational1/1 -> R/1

== system w3_warplab_trigger_proc/Trigger Sources/Ethernet B/Pkt Comp/Word Comp 1/Byte Comp 0/Equal ==
  D : Inport
  BT : Inport  Port=2
  Relational : xbsIndex_r4/Relational  mode=a=b  en=off  latency=0  dbl_ovrd=off  block_type=relational
  R : Outport
  wires:
  D/1 -> Relational/1
  BT/1 -> Relational/2
  Relational/1 -> R/1

== system w3_warplab_trigger_proc/Trigger Sources/Ethernet B/Pkt Comp/Word Comp 1/Byte Comp 0/Not Equal ==
  D : Inport
  BT : Inport  Port=2
  Relational : xbsIndex_r4/Relational  mode=a!=b  en=off  latency=0  dbl_ovrd=off  block_type=relational
  R : Outport
  wires:
  Relational/1 -> R/1
  BT/1 -> Relational/2
  D/1 -> Relational/1

== system w3_warplab_trigger_proc/Trigger Sources/Ethernet B/Pkt Comp/Word Comp 1/Byte Comp 1/Any of AND ==
  D : Inport
  T : Inport  Port=2
  Constant3 : xbsIndex_r4/Constant  const=0  gui_display_data_type=Fixed-point  arith_type=Unsigned  n_bits=8  bin_pt=0  preci_type=Single  exp_width=8  frac_width=24  explicit_period=off  period=1  equ=P=C  opselect=C  inp2=PCIN>>17  opr=+  inp1=P  carry=CIN  dbl_ovrd=off  block_type=constant
  Logical : xbsIndex_r4/Logical  logical_function=AND  inputs=2  en=off  latency=0  precision=Full  arith_type=Unsigned  n_bits=16  bin_pt=0  align_bp=on  dbl_ovrd=off  block_type=logical
  Relational1 : xbsIndex_r4/Relational  mode=a!=b  en=off  latency=0  dbl_ovrd=off  block_type=relational
  R : Outport
  wires:
  Relational1/1 -> R/1
  T/1 -> Logical/2
  D/1 -> Logical/1
  Logical/1 -> Relational1/2
  Constant3/1 -> Relational1/1

== system w3_warplab_trigger_proc/Trigger Sources/Ethernet B/Pkt Comp/Word Comp 1/Byte Comp 1/Equal ==
  D : Inport
  BT : Inport  Port=2
  Relational : xbsIndex_r4/Relational  mode=a=b  en=off  latency=0  dbl_ovrd=off  block_type=relational
  R : Outport
  wires:
  Relational/1 -> R/1
  BT/1 -> Relational/2
  D/1 -> Relational/1

== system w3_warplab_trigger_proc/Trigger Sources/Ethernet B/Pkt Comp/Word Comp 1/Byte Comp 1/Not Equal ==
  D : Inport
  BT : Inport  Port=2
  Relational : xbsIndex_r4/Relational  mode=a!=b  en=off  latency=0  dbl_ovrd=off  block_type=relational
  R : Outport
  wires:
  D/1 -> Relational/1
  BT/1 -> Relational/2
  Relational/1 -> R/1

== system w3_warplab_trigger_proc/Trigger Sources/Ethernet B/Pkt Comp/Word Comp 1/Byte Comp 2/Any of AND ==
  D : Inport
  T : Inport  Port=2
  Constant3 : xbsIndex_r4/Constant  const=0  gui_display_data_type=Fixed-point  arith_type=Unsigned  n_bits=8  bin_pt=0  preci_type=Single  exp_width=8  frac_width=24  explicit_period=off  period=1  equ=P=C  opselect=C  inp2=PCIN>>17  opr=+  inp1=P  carry=CIN  dbl_ovrd=off  block_type=constant
  Logical : xbsIndex_r4/Logical  logical_function=AND  inputs=2  en=off  latency=0  precision=Full  arith_type=Unsigned  n_bits=16  bin_pt=0  align_bp=on  dbl_ovrd=off  block_type=logical
  Relational1 : xbsIndex_r4/Relational  mode=a!=b  en=off  latency=0  dbl_ovrd=off  block_type=relational
  R : Outport
  wires:
  Constant3/1 -> Relational1/1
  Logical/1 -> Relational1/2
  D/1 -> Logical/1
  T/1 -> Logical/2
  Relational1/1 -> R/1
